simulink model "frictionmodel"  (R2018b)
settings: configuration reference "Physics" (kept outside this file)
model workspace (MAT data in the model file):
  veh_param = Simulink.Parameter
  veh_param.Value.cLiftF = 0
  veh_param.Value.cLiftR = 0
  veh_param.Value.CoGx_m = 0
  veh_param.Value.CoGy_m = 0
  veh_param.Value.CoGz_m = 0
  veh_param.Value.cDrag = 0
  veh_param.Value.Aref_m2 = 0
  veh_param.Value.Gearratio = 0
  veh_param.Value.Wheelbase_m = 0
  veh_param.Value.PacLatF = [0 0 0 0 0]
  veh_param.Value.PacLongF = [0 0 0 0 0]
  veh_param.Value.PacLatR = [0 0 0 0 0]
  veh_param.Value.PacLongR = [0 0 0 0 0]
  veh_param.Value.cRollFriction_Npmps = 0
  veh_param.Value.MaxRollFriction_N = 0
  veh_param.Value.T_YawRate_s = 0
  veh_param.Value.T_LatVel_s = 0
  veh_param.Value.TrackWidthF_m = 0
  veh_param.Value.TrackWidthR_m = 0
  veh_param.Value.TireRadiusF_m = 0
  veh_param.Value.TireRadiusR_m = 0
  veh_param.Value.VehicleInertia_kgm2 = 0
  veh_param.Value.WheelInertiaF_kgm2 = 0
  veh_param.Value.WheelInertiaR_kgm2 = 0
  veh_param.Value.VehicleMass_kg = 0
  veh_param.Value.switchModelBlend_mps = 0
  veh_param.Value.PTLimitLowVel_N = 0
  veh_param.Value.switchModelVel_mps = 0
  veh_param.Value.T_Tire_s = 0
  veh_param.DataType = 'struct'
  veh_param.Dimensions = [1 1]
  x0_positionstates = Simulink.Parameter
  x0_positionstates.Value = [0 0 0]
  x0_positionstates.DataType = 'auto'
  x0_positionstates.Dimensions = [1 3]
settings Model: DataDictionary=frictionmodel.sldd  OrderedModelArguments=off  Creator=wischnewski  LastModifiedBy=ga25xiw

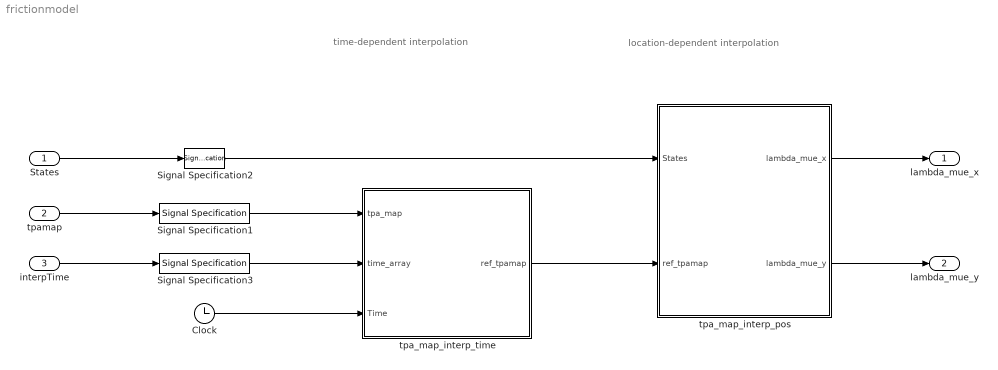
== system frictionmodel ==
  note: location-dependent interpolation
  note: time-dependent interpolation
  States : Inport
  tpamap : Inport  Port=2
  interpTime : Inport  Port=3
  Clock : Clock
  Signal Specification1 : SignalSpecification  Dimensions=[2500 23]
  Signal Specification2 : SignalSpecification  Dimensions=[1,2]
  Signal Specification3 : SignalSpecification  Dimensions=[1 10]
  tpa_map_interp_pos : MATLAB Function  TreatAsAtomicUnit=on
  tpa_map_interp_time : MATLAB Function  TreatAsAtomicUnit=on
  lambda_mue_x : Outport
  lambda_mue_y : Outport  Port=2
  wires:
  States/1 -> Signal Specification2/1
  Signal Specification2/1 -> tpa_map_interp_pos/1(States)
  tpa_map_interp_pos/1(lambda_mue_x) -> lambda_mue_x/1
  tpa_map_interp_pos/2(lambda_mue_y) -> lambda_mue_y/1
  tpa_map_interp_time/1(ref_tpamap) -> tpa_map_interp_pos/2(ref_tpamap)
  Clock/1 -> tpa_map_interp_time/3(Time)
  tpamap/1 -> Signal Specification1/1
  interpTime/1 -> Signal Specification3/1
  Signal Specification1/1 -> tpa_map_interp_time/1(tpa_map)
  Signal Specification3/1 -> tpa_map_interp_time/2(time_array)

== matlab function frictionmodel/tpa_map_interp_time ==
  data: tpa_map input; ref_tpamap output; time_array input; Time input
function ref_tpamap   = fcn(tpa_map, time_array, Time)

[ref_tpamap] = tpa_map_interp_time(tpa_map, time_array, Time);

== matlab function frictionmodel/tpa_map_interp_pos ==
  data: States input; lambda_mue_x output; lambda_mue_y output; ref_tpamap input
function [lambda_mue_x, lambda_mue_y]  = fcn(States, ref_tpamap)

[lambda_mue_x, lambda_mue_y] = tpa_map_interp_pos(States, ref_tpamap);
